simulink model "Poten1"  (R2024b)
settings: Solver=FixedStepAuto  StartTime=0.0  StopTime=10  FixedStep=0.01  RelTol=1e-3  EnableMultiTasking=on
libraries: stm32f4xxblockslib x1
settings Model: STM32="{\"AnalogInput\":{\"ID\":\"Poten1:1\"}}"  Creator=pongn  LastModifiedBy=pongn
settings OptimizationCC: DefaultParameterBehavior=Inlined  EnhancedBackFolding=on  PassReuseOutputArgsAs=Individual arguments  ZeroExternalMemoryAtStartup=off  ZeroInternalMemoryAtStartup=off  MaxStackSize=512  OptimizeBlockOrder=speed  DifferentSizesBufferReuse=on  OptimizationCustomize=off  EfficientTunableParamExpr=on
settings DebuggingCC: ParameterTunabilityLossMsg=error
settings HardwareCC: ProdBitPerPointer=32  ProdBitPerSizeT=32  ProdBitPerPtrDiffT=32  ProdLargestAtomicInteger=Long  ProdLargestAtomicFloat=Double  ProdWordSize=32  ProdLongLongMode=on  ProdHWDeviceType=ARM Compatible->ARM Cortex-M
settings SFSimCC: MATLABDynamicMemAlloc=off
settings RTWCC: Description=Embedded Coder  SystemTargetFile=ert.tlc  HardwareBoard=STM32G4xx Based  TemplateMakefile=ert_default_tmf  Toolchain=GNU Tools for ARM Embedded Processors
settings CodeAppCC: ForceParamTrailComments=on  IgnoreCustomStorageClasses=off  OperatorAnnotations=on  SimulinkDataObjDesc=on  SFDataObjDesc=on  InsertBlockDesc=on
settings ERTTargetCC: TargetLangStandard=C99 (ISO)  CodeReplacementLibrary=ARM Cortex-M  ExtModeTransport=3  ExtModeStaticAlloc=on  ExtModeStaticAllocSize=2048  ExtModeMexFile=ext_xcp  ExtModeIntrfLevel=Level2 - Open

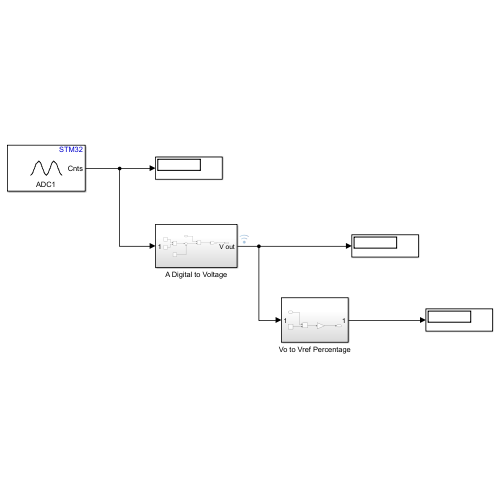
[thumbnail: Simulink's stored preview of the top-level diagram]
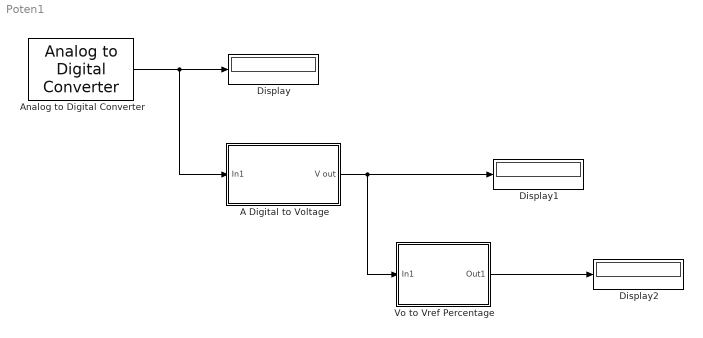
== system Poten1 ==
  A Digital to Voltage : Subsystem
  Analog to Digital Converter : stm32f4xxblockslib/Analog to Digital Converter  ADCModule=ADC1  ConversionGroup=Regular  TriggerMode=Trigger and read  NumberOfConversions=1  EnableBufferConv=off  BufferLength=1  OutputStatus=off  SampleTime=-1  EnableSimPort=off  hoistedMaskSrc=ECSoC/ECSimCodegen/Analog to Digital Converter
  Display : Display
  Display1 : Display
  Display2 : Display
  Vo to Vref Percentage : Subsystem
  wires:
  Analog to Digital Converter/1 -> A Digital to Voltage/1(In1), Display/1
  Vo to Vref Percentage/1(Out1) -> Display2/1
  A Digital to Voltage/1(V out) -> Display1/1, Vo to Vref Percentage/1(In1)

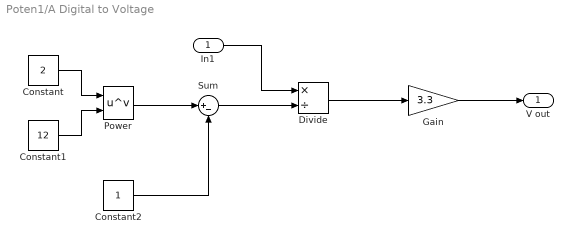
== system Poten1/A Digital to Voltage ==
  In1 : Inport
  Constant : Constant  Value=2
  Constant1 : Constant  Value=12
  Constant2 : Constant
  Divide : Product  Inputs=*/
  Gain : Gain  Gain=3.3
  Power : Math  Operator=pow
  Sum : Sum  Inputs=|+-
  V out : Outport
  wires:
  Constant/1 -> Power/1
  Constant2/1 -> Sum/2
  Sum/1 -> Divide/2
  Power/1 -> Sum/1
  Divide/1 -> Gain/1
  Constant1/1 -> Power/2
  Gain/1 -> V out/1
  In1/1 -> Divide/1

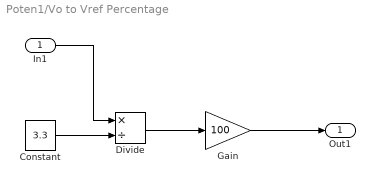
== system Poten1/Vo to Vref Percentage ==
  In1 : Inport
  Constant : Constant  Value=3.3
  Divide : Product  Inputs=*/
  Gain : Gain  Gain=100
  Out1 : Outport
  wires:
  Constant/1 -> Divide/2
  Divide/1 -> Gain/1
  In1/1 -> Divide/1
  Gain/1 -> Out1/1
